simulink model "prim_sec_tert_control"  (R2023b)
settings: Solver=VariableStepAuto  StartTime=0.0  StopTime=3000  RelTol=1e-3
settings Model: Creator=user  LastModifiedBy=user

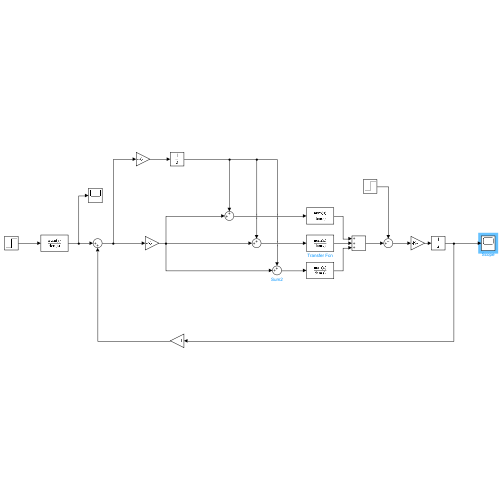
[thumbnail: Simulink's stored preview of the top-level diagram]
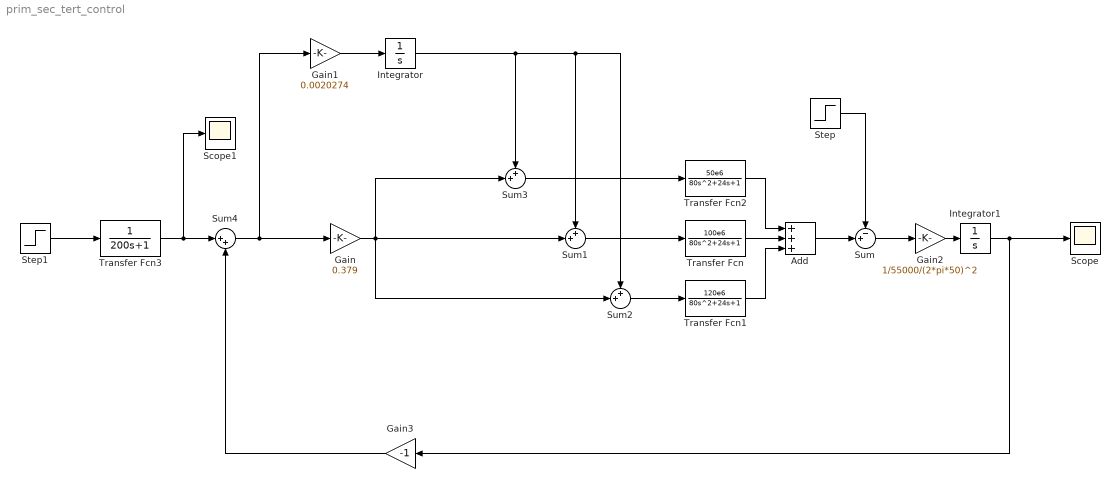
== system prim_sec_tert_control ==
  Add : Sum  Inputs=+++
  Gain : Gain  Gain=0.379
  Gain1 : Gain  Gain=0.0020274
  Gain2 : Gain  Gain=1/55000/(2*pi*50)^2
  Gain3 : Gain  Gain=-1
  Integrator : Integrator
  Integrator1 : Integrator
  Scope : Scope
  Scope1 : Scope
  Step : Step  Time=2000  After=30e6  SampleTime=0
  Step1 : Step  After=50  SampleTime=0
  Sum : Sum  Inputs=-+|
  Sum1 : Sum  Inputs=++|
  Sum2 : Sum  Inputs=++|
  Sum3 : Sum  Inputs=++|
  Sum4 : Sum  Inputs=|++
  Transfer Fcn : TransferFcn  Numerator=[100e6]  Denominator=[80 24 1]
  Transfer Fcn1 : TransferFcn  Numerator=[120e6]  Denominator=[80 24 1]
  Transfer Fcn2 : TransferFcn  Numerator=[50e6]  Denominator=[80 24 1]
  Transfer Fcn3 : TransferFcn  Denominator=[200 1]
  wires:
  Sum1/1 -> Transfer Fcn/1
  Step/1 -> Sum/1
  Gain1/1 -> Integrator/1
  Gain2/1 -> Integrator1/1
  Integrator1/1 -> Gain3/1, Scope/1
  Sum/1 -> Gain2/1
  Add/1 -> Sum/2
  Transfer Fcn/1 -> Add/2
  Transfer Fcn1/1 -> Add/3
  Transfer Fcn2/1 -> Add/1
  Sum2/1 -> Transfer Fcn1/1
  Sum3/1 -> Transfer Fcn2/1
  Gain/1 -> Sum3/2, Sum1/2, Sum2/2
  Integrator/1 -> Sum3/1, Sum2/1, Sum1/1
  Sum4/1 -> Gain1/1, Gain/1
  Gain3/1 -> Sum4/2
  Step1/1 -> Transfer Fcn3/1
  Transfer Fcn3/1 -> Scope1/1, Sum4/1
